simulink model "mcb_mech_param_est_host"  (R2023a)
settings: Solver=FixedStepDiscrete  StartTime=0.0  StopTime=inf  RelTol=1e-3  EnableMultiTasking=on
undefined symbols (not defined in the file): Ts_uart
libraries: instrumentseriallib x3, embeddedblockslib x1, simulink x1
settings Model: Creator=The MathWorks, Inc.  LastModifiedBy=snarayan
settings SolverCC: AlgebraicLoopSolver=TrustRegion
settings DataIOCC: LimitDataPoints=on  SaveFormat=Array  ReturnWorkspaceOutputs=off
settings OptimizationCC: LifeSpan=1  EfficientTunableParamExpr=on
settings DebuggingCC: MergeDetectMultiDrivingBlocksExec=none  SolverPrmCheckMsg=warning  ParameterPrecisionLossMsg=none  UnconnectedInputMsg=warning  UnconnectedOutputMsg=warning  UnconnectedLineMsg=warning  AllowSymbolicDim=off  PregeneratedLibrarySubsystemCodeDiagnostic=none  SFUnexpectedBacktrackingDiag=warning  SFNoUnconditionalDefaultTransitionDiag=warning  SFExecutionAtInitializationDiag=none  ArithmeticOperatorsInVariantConditions=warning
settings HardwareCC: ProdBitPerPointer=32  ProdLargestAtomicFloat=None  ProdIntDivRoundTo=Undefined  ProdEndianess=Unspecified  ProdWordSize=32  ProdHWDeviceType=32-bit Generic
settings ModelReferenceCC: EnableRefExpFcnMdlSchedulingChecks=on  PropagateSignalLabelsOutOfModel=off
settings SFSimCC: SimUseLocalCustomCode=off  MATLABDynamicMemAlloc=off
settings RTWCC: Description=Real-Time Workshop Embedded Coder  SystemTargetFile=ert.tlc  TemplateMakefile=ert_default_tmf  GenerateReport=on  RTWUseLocalCustomCode=off  IncludeHyperlinkInReport=on  LaunchReport=on  GenerateTraceInfo=on  GenerateTraceReport=on  GenerateTraceReportSl=on  GenerateTraceReportSf=on  GenerateTraceReportEml=on  DLArmComputeVersion=19.05
settings CodeAppCC: IgnoreCustomStorageClasses=off  StateflowObjectComments=on  InternalIdentifier=Classic
settings ERTTargetCC: MultiwordLength=2048  GenerateSampleERTMain=on  ERTCustomFileTemplate=example_file_process.tlc  ConvertIfToSwitch=off  SuppressUnreachableDefaultCases=off
settings ConfigComp: CovMetricSettings=dw  CovSaveCumulativeToWorkspaceVar=on  CovSaveSingleToWorkspaceVar=on  CovExternalEMLEnable=off  CovSFcnEnable=off

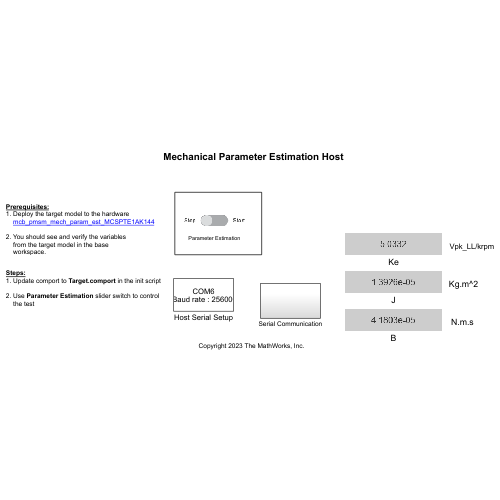
[thumbnail: Simulink's stored preview of the top-level diagram]
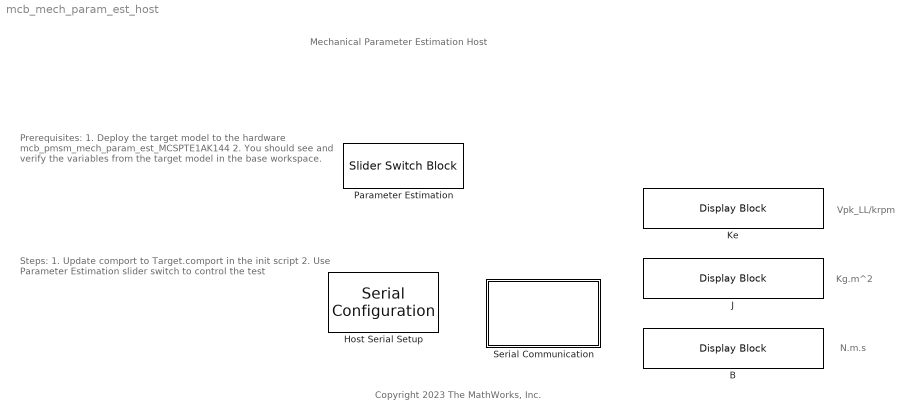
== system mcb_mech_param_est_host ==
  note: Mechanical Parameter Estimation Host
  note: Prerequisites:
      | 1. Deploy the target model to the hardware
      | mcb_pmsm_mech_param_est_MCSPTE1AK144
      |
      | 2. You should see and verify the variables
      | from the target model in the base
      | workspace.
  note: Copyright 2023 The MathWorks, Inc.
  note: Steps:
      | 1. Update comport to Target.comport in the init script
      |
      | 2. Use Parameter Estimation slider switch to control
      | the test
  note: N.m.s
  note: Kg.m^2
  note: Vpk_LL/krpm
  B : DisplayBlock  LabelPosition=Hide  Transparency=1
  Host Serial Setup : instrumentseriallib/Serial Configuration  Priority=-99  PortSel=Target.comport  Port=Target.comport   ComPort=Target.comport  BaudRate=256000  DataBits=8  Parity=none  StopBits=1  ByteOrder=little-endian  FlowControl=none  Timeout=2  SimulateUsing=Interpreted execution  BlockInModel=on  aMode=5
      settings: LibrarySourceBlock=mcbhostblockslib/Host Serial Setup
  J : DisplayBlock  LabelPosition=Hide  Transparency=1
  Ke : DisplayBlock  LabelPosition=Hide  Transparency=1
  Parameter Estimation : SliderSwitchBlock  LabelPosition=Hide
      settings: Values={{'Stop', 'Start'}, [0 1]}
  Serial Communication : Subsystem

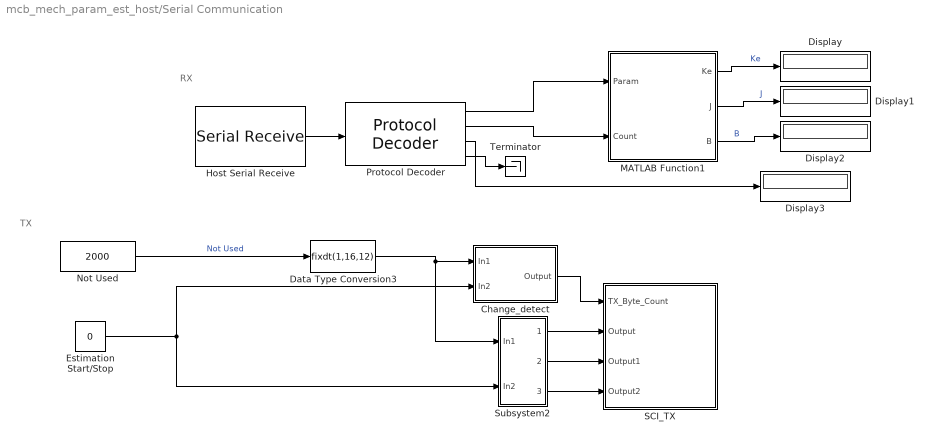
== system mcb_mech_param_est_host/Serial Communication ==
  note: RX
  note: TX
  Change_detect : Subsystem
  Data Type Conversion3 : DataTypeConversion  OutDataTypeStr=fixdt(1,16,12)  RndMeth=Simplest  SaturateOnIntegerOverflow=off
  Display{,1..3} (4 alike) : Display
  Estimation Start/Stop : Constant  Value=0  OutDataTypeStr=Inherit: Inherit via back propagation
  Host Serial Receive : instrumentseriallib/Serial Receive  PortSel=Target.comport  Port=Target.comport   ComPort=Target.comport  DataType=uint8  SaveDataType=uint8  ToggleHeader=off  Header='S'  ToggleTerminator=off  Terminator=Custom terminator  CustomTerminator='E'  InputFormat=Row major  ToggleDataSize=on  DataSize=7  EnableBlockingMode=on  ActionDataUnavailable=Output custom value  ActionWhenDataUnavailable=Output custom value  CustomValue=15  SampleTime=Ts_uart  SimulateUsing=Interpreted execution  BlockInModel=on  aMode=5
      settings: LibrarySourceBlock=mcbhostblockslib/Host Serial Receive
  MATLAB Function1 : MATLAB Function  TreatAsAtomicUnit=on
  Not Used : Constant  Value=2000  VectorParams1D=off  OutDataTypeStr=single  SampleTime=Ts_uart * 100
  Protocol Decoder : embeddedblockslib/Protocol Decoder  IsParseCSV=off  Header='S'  FieldTable={ 'Param', '1', 'single', 'Little endian'; 'Count', '1', 'uint8', 'Little endian'; 'Status', '1', 'uint8', 'Little endian' }  IsVariableSizeLastField=off  MaxVariableSizeFieldLength=[]  IsChecksumRequired=off  ChecksumAlgorithm=XOR of bytes  ChecksumSize=[]  TerminatorOption=<none>  CustomTerminatorVal=[]  IsInputLengthAvailable=off
      settings: LibrarySourceBlock=c2000lib/Target Communication/Protocol Decoder
  SCI_TX : Subsystem  TreatAsAtomicUnit=on
  Subsystem2 : Subsystem
  Terminator : Terminator
  wires:
  Estimation Start/Stop/1 -> Change_detect/2(In2), Subsystem2/2(In2)
  Not Used/1 -> Data Type Conversion3/1  "Not Used"
  Subsystem2/1(Output) -> SCI_TX/2(Output)
  Subsystem2/2(Output1) -> SCI_TX/3(Output1)
  Subsystem2/3(Output2) -> SCI_TX/4(Output2)
  Change_detect/1(Output) -> SCI_TX/1(TX_Byte_Count)
  Data Type Conversion3/1 -> Change_detect/1(In1), Subsystem2/1(In1)
  Host Serial Receive/1 -> Protocol Decoder/1
  Protocol Decoder/1 -> MATLAB Function1/1(Param)
  Protocol Decoder/2 -> MATLAB Function1/2(Count)
  Protocol Decoder/4 -> Terminator/1
  MATLAB Function1/1(Ke) -> Display/1  "Ke"
  MATLAB Function1/2(J) -> Display1/1  "J"
  MATLAB Function1/3(B) -> Display2/1  "B"
  Protocol Decoder/3 -> Display3/1

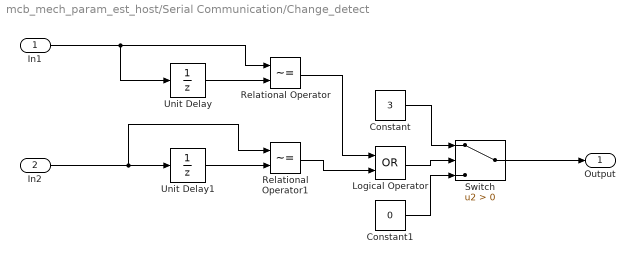
== system mcb_mech_param_est_host/Serial Communication/Change_detect ==
  In1 : Inport
  In2 : Inport  Port=2
  Constant : Constant  Value=3  OutDataTypeStr=uint8
  Constant1 : Constant  Value=0  OutDataTypeStr=uint8
  Logical Operator : Logic  Operator=OR  AllPortsSameDT=off  OutDataTypeStr=boolean
  Relational Operator : RelationalOperator  Operator=~=  OutDataTypeStr=boolean  InputSameDT=off
  Relational Operator1 : RelationalOperator  Operator=~=  OutDataTypeStr=boolean  InputSameDT=off
  Switch : Switch  Criteria=u2 > Threshold  SaturateOnIntegerOverflow=off  InputSameDT=off
  Unit Delay : UnitDelay  InitialCondition=0.5  SampleTime=-1  HasFrameUpgradeWarning=on
  Unit Delay1 : UnitDelay  SampleTime=-1  HasFrameUpgradeWarning=on
  Output : Outport
  wires:
  In2/1 -> Relational Operator1/1, Unit Delay1/1
  Unit Delay1/1 -> Relational Operator1/2
  Relational Operator1/1 -> Logical Operator/2
  Unit Delay/1 -> Relational Operator/2
  In1/1 -> Relational Operator/1, Unit Delay/1
  Relational Operator/1 -> Logical Operator/1
  Switch/1 -> Output/1
  Logical Operator/1 -> Switch/2
  Constant/1 -> Switch/1
  Constant1/1 -> Switch/3

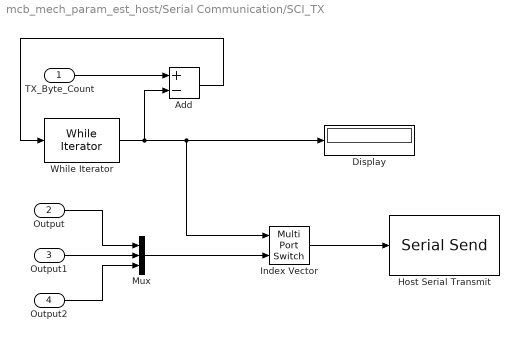
== system mcb_mech_param_est_host/Serial Communication/SCI_TX ==
  TX_Byte_Count : Inport
  Output : Inport  Port=2
  Output1 : Inport  Port=3
  Output2 : Inport  Port=4
  Add : Sum  Inputs=+-  OutDataTypeStr=Inherit: Same as first input
  Display : Display
  Host Serial Transmit : instrumentseriallib/Serial Send  PortSel=Target.comport  Port=Target.comport   ComPort=Target.comport  Header=[]  Terminator=<none>  CustomTerminator=[]  EnableBlockingMode=off  SimulateUsing=Interpreted execution  BlockInModel=on  aMode=5
      settings: LibrarySourceBlock=mcbhostblockslib/Host Serial Transmit
  Index Vector : MultiPortSwitch  Inputs=1  SaturateOnIntegerOverflow=off  InputSameDT=off
  Mux : Mux  Inputs=3
  While Iterator : WhileIterator  MaxIters=3  WhileBlockType=do-while  ShowIterationPort=on  OutputDataType=int16
  wires:
  Output/1 -> Mux/1
  Output2/1 -> Mux/3
  Output1/1 -> Mux/2
  Mux/1 -> Index Vector/2
  Index Vector/1 -> Host Serial Transmit/1
  TX_Byte_Count/1 -> Add/1
  Add/1 -> While Iterator/1
  While Iterator/1 -> Index Vector/1, Display/1, Add/2

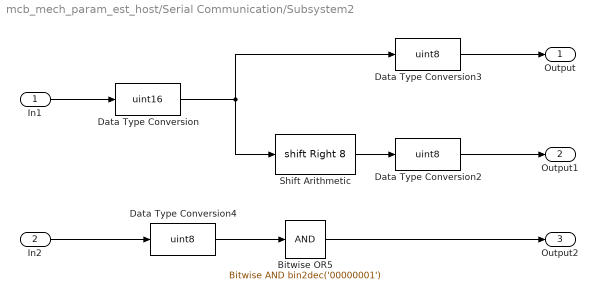
== system mcb_mech_param_est_host/Serial Communication/Subsystem2 ==
  In1 : Inport
  In2 : Inport  Port=2
  Bitwise OR5 : simulink/Logic and Bit Operations/Bitwise Operator  logicop=AND  UseBitMask=on  BitMask=bin2dec('00000001')  BitMaskRealWorld=Stored Integer
  Data Type Conversion : DataTypeConversion  OutDataTypeStr=uint16  ConvertRealWorld=Stored Integer (SI)  RndMeth=Simplest  SaturateOnIntegerOverflow=off
  Data Type Conversion2 : DataTypeConversion  OutDataTypeStr=uint8  ConvertRealWorld=Stored Integer (SI)  RndMeth=Simplest  SaturateOnIntegerOverflow=off
  Data Type Conversion3 : DataTypeConversion  OutDataTypeStr=uint8  ConvertRealWorld=Stored Integer (SI)  RndMeth=Simplest  SaturateOnIntegerOverflow=off
  Data Type Conversion4 : DataTypeConversion  OutDataTypeStr=uint8  ConvertRealWorld=Stored Integer (SI)  RndMeth=Simplest  SaturateOnIntegerOverflow=off
  Shift Arithmetic : ArithShift  BitShiftNumber=8  BitShiftDirection=Right
  Output : Outport
  Output1 : Outport  Port=2
  Output2 : Outport  Port=3
  wires:
  In1/1 -> Data Type Conversion/1
  Data Type Conversion/1 -> Shift Arithmetic/1, Data Type Conversion3/1
  Data Type Conversion4/1 -> Bitwise OR5/1
  Shift Arithmetic/1 -> Data Type Conversion2/1
  In2/1 -> Data Type Conversion4/1
  Data Type Conversion2/1 -> Output1/1
  Data Type Conversion3/1 -> Output/1
  Bitwise OR5/1 -> Output2/1

== matlab function mcb_mech_param_est_host/Serial Communication/MATLAB Function1 ==
  data: Ke output; J output; B output; Param input; Count input
function [ Ke, J, B] = unBuf(Param, Count)

persistent KeLocal;
if isempty(KeLocal)
KeLocal = single(0);
end

persistent JLocal;
if isempty(JLocal)
JLocal = single(0);
end

persistent BLocal;
if isempty(BLocal)
BLocal = single(0);
end

if (Count ==1)
    KeLocal = Param;
elseif (Count ==2)
    JLocal = Param;
elseif (Count ==3)
    BLocal = Param;
end

Ke = KeLocal;
J = JLocal;
B = BLocal;
end
